simulink library "SEN_SSS"  (Simulink 10.2)
settings: Solver=VariableStepAuto  StartTime=0.0  StopTime=10.0  RelTol=1e-3
undefined symbols (not defined in the file): SEN_SSS_par
libraries: LIB_ROT x2, simulink x1, LIB_SEN x1
settings Model: Creator=dbell44  LastModifiedBy=dbell44

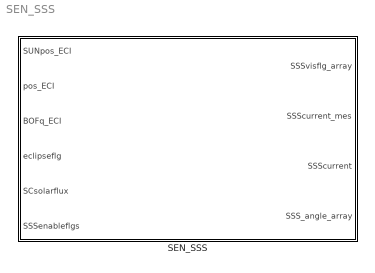
== system SEN_SSS ==
  SEN_SSS : Subsystem

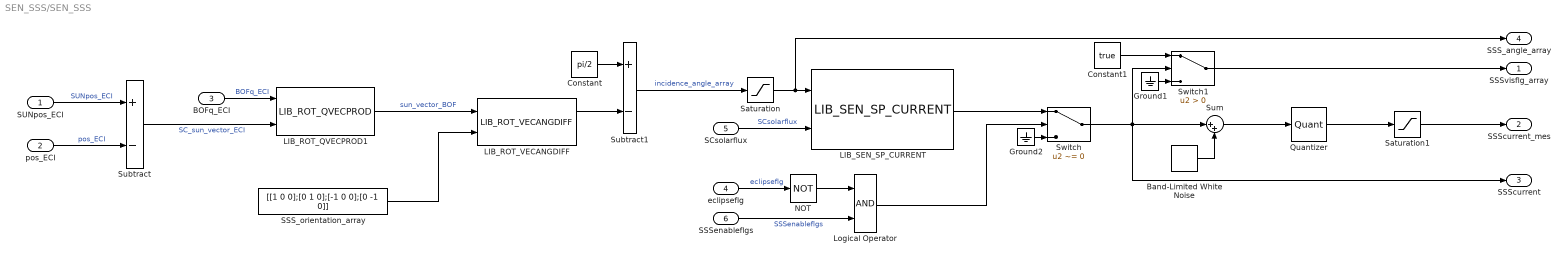
== system SEN_SSS/SEN_SSS ==
  SUNpos_ECI : Inport
  pos_ECI : Inport  Port=2
  BOFq_ECI : Inport  Port=3
  eclipseflg : Inport  Port=4
  SCsolarflux : Inport  Port=5
  SSSenableflgs : Inport  Port=6
  Band-Limited White Noise : simulink/Sources/Band-Limited White Noise  Cov=SEN_SSS_par.noise_power  Ts=1/SEN_SSS_par.sample_rate  seed=randi([1 243453])
  Constant : Constant  Value=pi/2
  Constant1 : Constant  Value=true
  Ground1 : Ground
  Ground2 : Ground
  LIB_ROT_QVECPROD1 : LIB_ROT/LIB_ROT_QVECPROD
  LIB_ROT_VECANGDIFF : LIB_ROT/LIB_ROT_VECANGDIFF  zero_tol=0
  LIB_SEN_SP_CURRENT : LIB_SEN/LIB_SEN_SP_CURRENT  eff=1  A=[1 1 1 1]  V=5
  Logical Operator : Logic  AllPortsSameDT=off  OutDataTypeStr=boolean
  NOT : Logic  Operator=NOT  IconShape=distinctive  AllPortsSameDT=off  OutDataTypeStr=boolean
  Quantizer : Quantizer  QuantizationInterval=SEN_SSS_par.sensitivity  LinearizeAsGain=off
  SSS_orientation_array : Constant  Value=[[1 0 0];[0 1 0];[-1 0 0];[0 -1 0]]
  Saturation : Saturate  UpperLimit=inf  LowerLimit=0
  Saturation1 : Saturate  UpperLimit=SEN_SSS_par.full_scale_range  LowerLimit=-SEN_SSS_par.full_scale_range
  Subtract : Sum  Inputs=+-
  Subtract1 : Sum  Inputs=+-
  Sum : Sum  Inputs=|++
  Switch : Switch  Criteria=u2 ~= 0
  Switch1 : Switch  Criteria=u2 > Threshold
  SSSvisflg_array : Outport  VectorParamsAs1DForOutWhenUnconnected=off
  SSScurrent_mes : Outport  Port=2  VectorParamsAs1DForOutWhenUnconnected=off
  SSScurrent : Outport  Port=3  VectorParamsAs1DForOutWhenUnconnected=off
  SSS_angle_array : Outport  Port=4  VectorParamsAs1DForOutWhenUnconnected=off
  wires:
  pos_ECI/1 -> Subtract/2  "pos_ECI"
  SUNpos_ECI/1 -> Subtract/1  "SUNpos_ECI"
  Subtract/1 -> LIB_ROT_QVECPROD1/2  "SC_sun_vector_ECI"
  BOFq_ECI/1 -> LIB_ROT_QVECPROD1/1  "BOFq_ECI"
  LIB_ROT_QVECPROD1/1 -> LIB_ROT_VECANGDIFF/1  "sun_vector_BOF"
  SSS_orientation_array/1 -> LIB_ROT_VECANGDIFF/2
  LIB_ROT_VECANGDIFF/1 -> Subtract1/2
  Constant/1 -> Subtract1/1
  Subtract1/1 -> Saturation/1  "incidence_angle_array"
  SCsolarflux/1 -> LIB_SEN_SP_CURRENT/2  "SCsolarflux"
  eclipseflg/1 -> NOT/1  "eclipseflg"
  SSSenableflgs/1 -> Logical Operator/2  "SSSenableflgs"
  Saturation/1 -> SSS_angle_array/1, LIB_SEN_SP_CURRENT/1
  NOT/1 -> Logical Operator/1
  Logical Operator/1 -> Switch/2
  LIB_SEN_SP_CURRENT/1 -> Switch/1
  Ground2/1 -> Switch/3
  Switch/1 -> Sum/1, SSScurrent/1, Switch1/2
  Ground1/1 -> Switch1/3
  Constant1/1 -> Switch1/1
  Switch1/1 -> SSSvisflg_array/1
  Band-Limited White Noise/1 -> Sum/2
  Sum/1 -> Quantizer/1
  Quantizer/1 -> Saturation1/1
  Saturation1/1 -> SSScurrent_mes/1
